simulink model "kurtosis_central_moment_calc"  (R2012b)
settings: Solver=ode45  StartTime=0.0  StopTime=199  RelTol=1e-3
libraries: xbsIndex_r4 x93, simulink_xsg_bridge x1
settings Model: Creator=sgowda  LastModifiedBy=sgowda

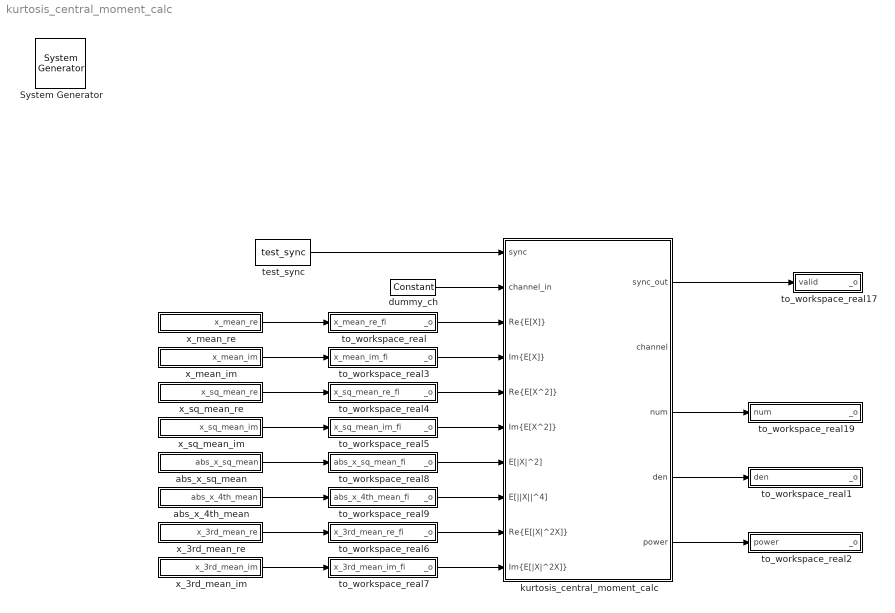
== system kurtosis_central_moment_calc ==
  " System Generator" : xbsIndex_r4/ System Generator  Tag=genX  xilinxfamily=Kintex7  part=xc7k325t  speed=-3  package=fbg676  synthesis_tool=XST  clock_wrapper=Clock Enables  directory=./netlist  proj_type=Project Navigator  Synth_file=XST Defaults  Impl_file=ISE Defaults  testbench=off  simulink_period=1  sysclk_period=10  dcm_input_clock_period=10  incr_netlist=off  trim_vbits=Everywhere in SubSystem  dbl_ovrd=According to Block Masks  core_generation=According to Block Masks  run_coregen=off  deprecated_control=off  eval_field=0  block_type=sysgen
  abs_x_4th_mean : Subsystem  mask{var_name=abs_x_4th_mean, n_bits=88, bin_pt=82, quantization=Round  (unbiased: +/- Inf), overflow=Saturate, arith_type=Signed  (2's comp)}
      mask prompts: var_name "Workspace variable name"; n_bits "# of bits"; bin_pt "Binary Point"; arith_type "Arithmetic type"
      mask init:
      | config.source = str2func('mat_input_data_init_xblock');
      | config.toplevel = gcb();
      | xBlock(config, {config.toplevel, 'var_name', var_name, ...
      |     'n_bits', n_bits, 'bin_pt', bin_pt, 'quantization', quantization, ...
      |     'overflow', overflow, 'arith_type', arith_type});
      mask TypeOptions quantization: Truncate | Round  (unbiased: +/- Inf) | Round  (unbiased: Even Values)
      mask TypeOptions overflow: Wrap | Saturate | Flag as error
      mask TypeOptions arith_type: Signed  (2's comp) | Boolean | Unsigned
  abs_x_sq_mean : Subsystem  mask{var_name=abs_x_sq_mean, n_bits=51, bin_pt=48, quantization=Round  (unbiased: +/- Inf), overflow=Saturate, arith_type=Signed  (2's comp)}
      mask prompts: var_name "Workspace variable name"; n_bits "# of bits"; bin_pt "Binary Point"; arith_type "Arithmetic type"
      mask init: same as kurtosis_central_moment_calc/abs_x_4th_mean
      mask TypeOptions quantization: Truncate | Round  (unbiased: +/- Inf) | Round  (unbiased: Even Values)
      mask TypeOptions overflow: Wrap | Saturate | Flag as error
      mask TypeOptions arith_type: Signed  (2's comp) | Boolean | Unsigned
  dummy_ch : xbsIndex_r4/Constant  const=1  gui_display_data_type=Fixed-point  arith_type=Signed (2's comp)  n_bits=16  bin_pt=14  preci_type=Single  exp_width=8  frac_width=24  explicit_period=on  period=1  equ=P=C  opselect=C  inp2=PCIN>>17  opr=+  inp1=P  carry=CIN  dbl_ovrd=off  block_type=constant
  kurtosis_central_moment_calc : Subsystem
  test_sync : simulink_xsg_bridge/test_sync
  to_workspace_real : Subsystem  mask{var_name=x_mean_re_fi}
      mask prompts: var_name "Workspace variable name"
      mask init:
      | config.source = str2func('mat_output_data_init_xblock');
      | config.toplevel = gcb();
      | xBlock(config, {config.toplevel, 'var_name', var_name});
  to_workspace_real1 : Subsystem  mask{var_name=den}
      mask prompts: var_name "Workspace variable name"
      mask init:
      | config.source = str2func('mat_output_data_init_xblock');
      | config.toplevel = gcb();
      | xBlock(config, {config.toplevel, 'var_name', var_name});
  to_workspace_real17 : Subsystem  mask{var_name=valid}
      mask prompts: var_name "Workspace variable name"
      mask init:
      | config.source = str2func('mat_output_data_init_xblock');
      | config.toplevel = gcb();
      | xBlock(config, {config.toplevel, 'var_name', var_name});
  to_workspace_real19 : Subsystem  mask{var_name=num}
      mask prompts: var_name "Workspace variable name"
      mask init:
      | config.source = str2func('mat_output_data_init_xblock');
      | config.toplevel = gcb();
      | xBlock(config, {config.toplevel, 'var_name', var_name});
  to_workspace_real2 : Subsystem  mask{var_name=power}
      mask prompts: var_name "Workspace variable name"
      mask init:
      | config.source = str2func('mat_output_data_init_xblock');
      | config.toplevel = gcb();
      | xBlock(config, {config.toplevel, 'var_name', var_name});
  to_workspace_real3 : Subsystem  mask{var_name=x_mean_im_fi}
      mask prompts: var_name "Workspace variable name"
      mask init:
      | config.source = str2func('mat_output_data_init_xblock');
      | config.toplevel = gcb();
      | xBlock(config, {config.toplevel, 'var_name', var_name});
  to_workspace_real4 : Subsystem  mask{var_name=x_sq_mean_re_fi}
      mask prompts: var_name "Workspace variable name"
      mask init:
      | config.source = str2func('mat_output_data_init_xblock');
      | config.toplevel = gcb();
      | xBlock(config, {config.toplevel, 'var_name', var_name});
  to_workspace_real5 : Subsystem  mask{var_name=x_sq_mean_im_fi}
      mask prompts: var_name "Workspace variable name"
      mask init:
      | config.source = str2func('mat_output_data_init_xblock');
      | config.toplevel = gcb();
      | xBlock(config, {config.toplevel, 'var_name', var_name});
  to_workspace_real6 : Subsystem  mask{var_name=x_3rd_mean_re_fi}
      mask prompts: var_name "Workspace variable name"
      mask init:
      | config.source = str2func('mat_output_data_init_xblock');
      | config.toplevel = gcb();
      | xBlock(config, {config.toplevel, 'var_name', var_name});
  to_workspace_real7 : Subsystem  mask{var_name=x_3rd_mean_im_fi}
      mask prompts: var_name "Workspace variable name"
      mask init:
      | config.source = str2func('mat_output_data_init_xblock');
      | config.toplevel = gcb();
      | xBlock(config, {config.toplevel, 'var_name', var_name});
  to_workspace_real8 : Subsystem  mask{var_name=abs_x_sq_mean_fi}
      mask prompts: var_name "Workspace variable name"
      mask init:
      | config.source = str2func('mat_output_data_init_xblock');
      | config.toplevel = gcb();
      | xBlock(config, {config.toplevel, 'var_name', var_name});
  to_workspace_real9 : Subsystem  mask{var_name=abs_x_4th_mean_fi}
      mask prompts: var_name "Workspace variable name"
      mask init:
      | config.source = str2func('mat_output_data_init_xblock');
      | config.toplevel = gcb();
      | xBlock(config, {config.toplevel, 'var_name', var_name});
  x_3rd_mean_im : Subsystem  mask{var_name=x_3rd_mean_im, n_bits=69, bin_pt=65, quantization=Round  (unbiased: +/- Inf), overflow=Saturate, arith_type=Signed  (2's comp)}
      mask prompts: var_name "Workspace variable name"; n_bits "# of bits"; bin_pt "Binary Point"; arith_type "Arithmetic type"
      mask init: same as kurtosis_central_moment_calc/abs_x_4th_mean
      mask TypeOptions quantization: Truncate | Round  (unbiased: +/- Inf) | Round  (unbiased: Even Values)
      mask TypeOptions overflow: Wrap | Saturate | Flag as error
      mask TypeOptions arith_type: Signed  (2's comp) | Boolean | Unsigned
  x_3rd_mean_re : Subsystem  mask{var_name=x_3rd_mean_re, n_bits=69, bin_pt=65, quantization=Round  (unbiased: +/- Inf), overflow=Saturate, arith_type=Signed  (2's comp)}
      mask prompts: var_name "Workspace variable name"; n_bits "# of bits"; bin_pt "Binary Point"; arith_type "Arithmetic type"
      mask init: same as kurtosis_central_moment_calc/abs_x_4th_mean
      mask TypeOptions quantization: Truncate | Round  (unbiased: +/- Inf) | Round  (unbiased: Even Values)
      mask TypeOptions overflow: Wrap | Saturate | Flag as error
      mask TypeOptions arith_type: Signed  (2's comp) | Boolean | Unsigned
  x_mean_im : Subsystem  mask{var_name=x_mean_im, n_bits=32, bin_pt=31, quantization=Round  (unbiased: +/- Inf), overflow=Saturate, arith_type=Signed  (2's comp)}
      mask prompts: var_name "Workspace variable name"; n_bits "# of bits"; bin_pt "Binary Point"; arith_type "Arithmetic type"
      mask init: same as kurtosis_central_moment_calc/abs_x_4th_mean
      mask TypeOptions quantization: Truncate | Round  (unbiased: +/- Inf) | Round  (unbiased: Even Values)
      mask TypeOptions overflow: Wrap | Saturate | Flag as error
      mask TypeOptions arith_type: Signed  (2's comp) | Boolean | Unsigned
  x_mean_re : Subsystem  mask{var_name=x_mean_re, n_bits=32, bin_pt=31, quantization=Round  (unbiased: +/- Inf), overflow=Saturate, arith_type=Signed  (2's comp)}
      mask prompts: var_name "Workspace variable name"; n_bits "# of bits"; bin_pt "Binary Point"; arith_type "Arithmetic type"
      mask init: same as kurtosis_central_moment_calc/abs_x_4th_mean
      mask TypeOptions quantization: Truncate | Round  (unbiased: +/- Inf) | Round  (unbiased: Even Values)
      mask TypeOptions overflow: Wrap | Saturate | Flag as error
      mask TypeOptions arith_type: Signed  (2's comp) | Boolean | Unsigned
  x_sq_mean_im : Subsystem  mask{var_name=x_sq_mean_im, n_bits=51, bin_pt=48, quantization=Round  (unbiased: +/- Inf), overflow=Saturate, arith_type=Signed  (2's comp)}
      mask prompts: var_name "Workspace variable name"; n_bits "# of bits"; bin_pt "Binary Point"; arith_type "Arithmetic type"
      mask init: same as kurtosis_central_moment_calc/abs_x_4th_mean
      mask TypeOptions quantization: Truncate | Round  (unbiased: +/- Inf) | Round  (unbiased: Even Values)
      mask TypeOptions overflow: Wrap | Saturate | Flag as error
      mask TypeOptions arith_type: Signed  (2's comp) | Boolean | Unsigned
  x_sq_mean_re : Subsystem  mask{var_name=x_sq_mean_re, n_bits=51, bin_pt=48, quantization=Round  (unbiased: +/- Inf), overflow=Saturate, arith_type=Signed  (2's comp)}
      mask prompts: var_name "Workspace variable name"; n_bits "# of bits"; bin_pt "Binary Point"; arith_type "Arithmetic type"
      mask init: same as kurtosis_central_moment_calc/abs_x_4th_mean
      mask TypeOptions quantization: Truncate | Round  (unbiased: +/- Inf) | Round  (unbiased: Even Values)
      mask TypeOptions overflow: Wrap | Saturate | Flag as error
      mask TypeOptions arith_type: Signed  (2's comp) | Boolean | Unsigned
  wires:
  test_sync/1 -> kurtosis_central_moment_calc/1(sync)
  kurtosis_central_moment_calc/1(sync_out) -> to_workspace_real17/1(valid)
  abs_x_sq_mean/1(abs_x_sq_mean) -> to_workspace_real8/1(abs_x_sq_mean_fi)
  x_mean_im/1(x_mean_im) -> to_workspace_real3/1(x_mean_im_fi)
  x_sq_mean_re/1(x_sq_mean_re) -> to_workspace_real4/1(x_sq_mean_re_fi)
  x_sq_mean_im/1(x_sq_mean_im) -> to_workspace_real5/1(x_sq_mean_im_fi)
  abs_x_4th_mean/1(abs_x_4th_mean) -> to_workspace_real9/1(abs_x_4th_mean_fi)
  x_3rd_mean_re/1(x_3rd_mean_re) -> to_workspace_real6/1(x_3rd_mean_re_fi)
  x_3rd_mean_im/1(x_3rd_mean_im) -> to_workspace_real7/1(x_3rd_mean_im_fi)
  kurtosis_central_moment_calc/3(num) -> to_workspace_real19/1(num)
  kurtosis_central_moment_calc/4(den) -> to_workspace_real1/1(den)
  kurtosis_central_moment_calc/5(power) -> to_workspace_real2/1(power)
  dummy_ch/1 -> kurtosis_central_moment_calc/2(channel_in)
  x_mean_re/1(x_mean_re) -> to_workspace_real/1(x_mean_re_fi)
  to_workspace_real/1(_o) -> kurtosis_central_moment_calc/3("Re{E[X]}")
  to_workspace_real3/1(_o) -> kurtosis_central_moment_calc/4("Im{E[X]}")
  to_workspace_real4/1(_o) -> kurtosis_central_moment_calc/5("Re{E[X^2]}")
  to_workspace_real5/1(_o) -> kurtosis_central_moment_calc/6("Im{E[X^2]}")
  to_workspace_real6/1(_o) -> kurtosis_central_moment_calc/9("Re{E[|X|^2X]}")
  to_workspace_real7/1(_o) -> kurtosis_central_moment_calc/10("Im{E[|X|^2X]}")
  to_workspace_real8/1(_o) -> kurtosis_central_moment_calc/7(E[|X|^2])
  to_workspace_real9/1(_o) -> kurtosis_central_moment_calc/8(E[||X||^4])

== system kurtosis_central_moment_calc/abs_x_4th_mean ==
  gateway : xbsIndex_r4/Gateway In  gui_display_data_type=Fixed-point  arith_type="Signed  (2's comp)"  n_bits=88  bin_pt=82  preci_type=Single  exp_width=8  frac_width=24  quantization="Round  (unbiased: +/- Inf)"  overflow=Saturate  period=1  dbl_ovrd=off  timing_constraint=None  locs_specified=off  LOCs={}  UseAsADC=off  ADCChannel='1'  inherit_from_input=off  hdl_port=on  block_type=gatewayin
  workspace_var : FromWorkspace  VariableName=abs_x_4th_mean  SampleTime=0
  abs_x_4th_mean : Outport
  wires:
  gateway/1 -> abs_x_4th_mean/1
  workspace_var/1 -> gateway/1

== system kurtosis_central_moment_calc/abs_x_sq_mean ==
  gateway : xbsIndex_r4/Gateway In  gui_display_data_type=Fixed-point  arith_type="Signed  (2's comp)"  n_bits=51  bin_pt=48  preci_type=Single  exp_width=8  frac_width=24  quantization="Round  (unbiased: +/- Inf)"  overflow=Saturate  period=1  dbl_ovrd=off  timing_constraint=None  locs_specified=off  LOCs={}  UseAsADC=off  ADCChannel='1'  inherit_from_input=off  hdl_port=on  block_type=gatewayin
  workspace_var : FromWorkspace  VariableName=abs_x_sq_mean  SampleTime=0
  abs_x_sq_mean : Outport
  wires:
  gateway/1 -> abs_x_sq_mean/1
  workspace_var/1 -> gateway/1

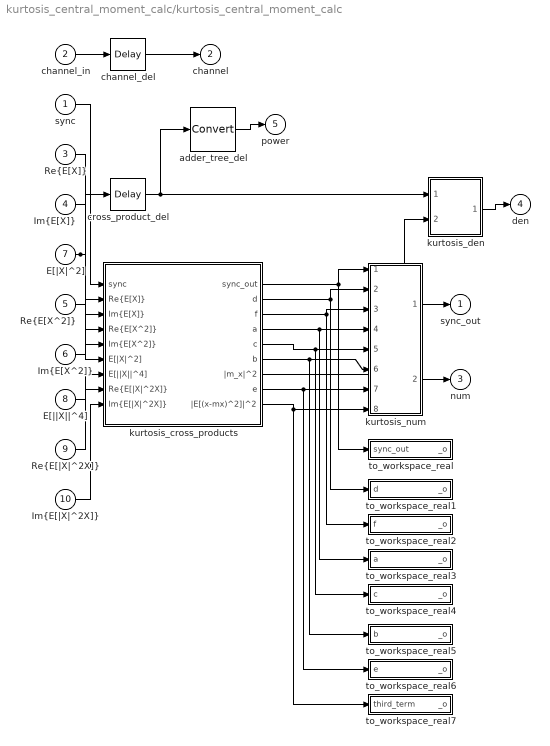
== system kurtosis_central_moment_calc/kurtosis_central_moment_calc ==
  sync : Inport
  channel_in : Inport  Port=2
  "Re{E[X]}" : Inport  Port=3
  "Im{E[X]}" : Inport  Port=4
  "Re{E[X^2]}" : Inport  Port=5
  "Im{E[X^2]}" : Inport  Port=6
  E[|X|^2] : Inport  Port=7
  E[||X||^4] : Inport  Port=8
  "Re{E[|X|^2X]}" : Inport  Port=9
  "Im{E[|X|^2X]}" : Inport  Port=10
  adder_tree_del : xbsIndex_r4/Convert  gui_display_data_type=Fixed-point  arith_type="Signed  (2's comp)"  n_bits=32  bin_pt=29  float_type=Single  exp_bits=8  fraction_bits=24  quantization="Round  (unbiased: +/- Inf)"  overflow=Saturate  en=off  latency=13  dbl_ovrd=off  pipeline=off  block_type=convert
  channel_del : xbsIndex_r4/Delay  rst=off  infoeditControl=Selection of Reset will increase slice count due to use of real FFs and instead of SRLs  en=off  latency=38  dbl_ovrd=off  reg_retiming=off  block_type=delay
  cross_product_del : xbsIndex_r4/Delay  rst=off  infoeditControl=Selection of Reset will increase slice count due to use of real FFs and instead of SRLs  en=off  latency=25  dbl_ovrd=off  reg_retiming=off  block_type=delay
  kurtosis_cross_products : Subsystem
  kurtosis_den : Subsystem
  kurtosis_num : Subsystem
  to_workspace_real : Subsystem  mask{var_name=sync_out}
      mask prompts: var_name "Workspace variable name"
      mask init:
      | config.source = str2func('mat_output_data_init_xblock');
      | config.toplevel = gcb();
      | xBlock(config, {config.toplevel, 'var_name', var_name});
  to_workspace_real1 : Subsystem  mask{var_name=d}
      mask prompts: var_name "Workspace variable name"
      mask init:
      | config.source = str2func('mat_output_data_init_xblock');
      | config.toplevel = gcb();
      | xBlock(config, {config.toplevel, 'var_name', var_name});
  to_workspace_real2 : Subsystem  mask{var_name=f}
      mask prompts: var_name "Workspace variable name"
      mask init:
      | config.source = str2func('mat_output_data_init_xblock');
      | config.toplevel = gcb();
      | xBlock(config, {config.toplevel, 'var_name', var_name});
  to_workspace_real3 : Subsystem  mask{var_name=a}
      mask prompts: var_name "Workspace variable name"
      mask init:
      | config.source = str2func('mat_output_data_init_xblock');
      | config.toplevel = gcb();
      | xBlock(config, {config.toplevel, 'var_name', var_name});
  to_workspace_real4 : Subsystem  mask{var_name=c}
      mask prompts: var_name "Workspace variable name"
      mask init:
      | config.source = str2func('mat_output_data_init_xblock');
      | config.toplevel = gcb();
      | xBlock(config, {config.toplevel, 'var_name', var_name});
  to_workspace_real5 : Subsystem  mask{var_name=b}
      mask prompts: var_name "Workspace variable name"
      mask init:
      | config.source = str2func('mat_output_data_init_xblock');
      | config.toplevel = gcb();
      | xBlock(config, {config.toplevel, 'var_name', var_name});
  to_workspace_real6 : Subsystem  mask{var_name=e}
      mask prompts: var_name "Workspace variable name"
      mask init:
      | config.source = str2func('mat_output_data_init_xblock');
      | config.toplevel = gcb();
      | xBlock(config, {config.toplevel, 'var_name', var_name});
  to_workspace_real7 : Subsystem  mask{var_name=third_term}
      mask prompts: var_name "Workspace variable name"
      mask init:
      | config.source = str2func('mat_output_data_init_xblock');
      | config.toplevel = gcb();
      | xBlock(config, {config.toplevel, 'var_name', var_name});
  sync_out : Outport
  channel : Outport  Port=2
  num : Outport  Port=3
  den : Outport  Port=4
  power : Outport  Port=5
  wires:
  E[|X|^2]/1 -> kurtosis_cross_products/6(E[|X|^2]), cross_product_del/1
  cross_product_del/1 -> kurtosis_den/1(E[|X|^2]), adder_tree_del/1
  channel_del/1 -> channel/1
  channel_in/1 -> channel_del/1
  kurtosis_num/2(E[|X-m_x|^4]) -> num/1
  kurtosis_num/1(sync_out) -> sync_out/1
  kurtosis_cross_products/9(|E[(x-mx)^2]|^2) -> to_workspace_real7/1(third_term), kurtosis_num/8(|E[(x-mx)^2]|^2)
  kurtosis_cross_products/8(e) -> to_workspace_real6/1(e), kurtosis_num/7(|m_x|^4)
  kurtosis_cross_products/6(b) -> to_workspace_real5/1(b), kurtosis_num/6("Re{4E[X|X|^2*m_x]}")
  kurtosis_cross_products/5(c) -> to_workspace_real4/1(c), kurtosis_num/5("Re{2E[X^2*conj(m_x^2)]}")
  kurtosis_cross_products/4(a) -> to_workspace_real3/1(a), kurtosis_num/4(E[|X|^4])
  kurtosis_cross_products/3(f) -> kurtosis_num/3(4|m_x|^4), to_workspace_real2/1(f)
  kurtosis_cross_products/2(d) -> kurtosis_num/2(4E[|X|^2]|m_x|^2), to_workspace_real1/1(d)
  kurtosis_cross_products/1(sync_out) -> kurtosis_num/1(sync), to_workspace_real/1(sync_out)
  kurtosis_den/1(E[|X-m_x|^2]^2) -> den/1
  kurtosis_cross_products/7(|m_x|^2) -> kurtosis_den/2(|m_x|^2)
  "Im{E[|X|^2X]}"/1 -> kurtosis_cross_products/9("Im{E[|X|^2X]}")
  "Re{E[|X|^2X]}"/1 -> kurtosis_cross_products/8("Re{E[|X|^2X]}")
  E[||X||^4]/1 -> kurtosis_cross_products/7(E[||X||^4])
  "Im{E[X^2]}"/1 -> kurtosis_cross_products/5("Im{E[X^2]}")
  "Re{E[X^2]}"/1 -> kurtosis_cross_products/4("Re{E[X^2]}")
  "Im{E[X]}"/1 -> kurtosis_cross_products/3("Im{E[X]}")
  "Re{E[X]}"/1 -> kurtosis_cross_products/2("Re{E[X]}")
  sync/1 -> kurtosis_cross_products/1(sync)
  adder_tree_del/1 -> power/1

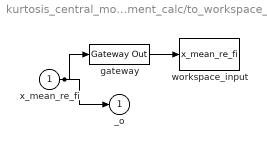
== system kurtosis_central_moment_calc/to_workspace_real ==
  x_mean_re_fi : Inport
  gateway : xbsIndex_r4/Gateway Out  inherit_from_input=on  hdl_port=off  timing_constraint=None  locs_specified=off  LOCs={}  UseAsDAC=off  DACChannel='1'  block_type=gatewayout
  workspace_input : ToWorkspace  VariableName=x_mean_re_fi  SampleTime=-1
  _o : Outport
  wires:
  x_mean_re_fi/1 -> gateway/1, _o/1
  gateway/1 -> workspace_input/1

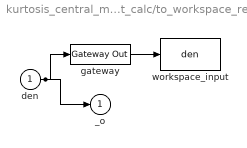
== system kurtosis_central_moment_calc/to_workspace_real1 ==
  den : Inport
  gateway : xbsIndex_r4/Gateway Out  inherit_from_input=on  hdl_port=off  timing_constraint=None  locs_specified=off  LOCs={}  UseAsDAC=off  DACChannel='1'  block_type=gatewayout
  workspace_input : ToWorkspace  VariableName=den  SampleTime=-1
  _o : Outport
  wires:
  den/1 -> gateway/1, _o/1
  gateway/1 -> workspace_input/1

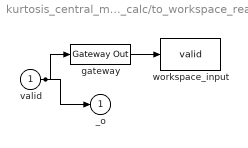
== system kurtosis_central_moment_calc/to_workspace_real17 ==
  valid : Inport
  gateway : xbsIndex_r4/Gateway Out  inherit_from_input=on  hdl_port=off  timing_constraint=None  locs_specified=off  LOCs={}  UseAsDAC=off  DACChannel='1'  block_type=gatewayout
  workspace_input : ToWorkspace  VariableName=valid  SampleTime=-1
  _o : Outport
  wires:
  valid/1 -> gateway/1, _o/1
  gateway/1 -> workspace_input/1

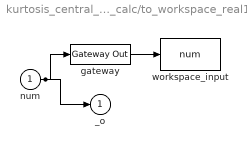
== system kurtosis_central_moment_calc/to_workspace_real19 ==
  num : Inport
  gateway : xbsIndex_r4/Gateway Out  inherit_from_input=on  hdl_port=off  timing_constraint=None  locs_specified=off  LOCs={}  UseAsDAC=off  DACChannel='1'  block_type=gatewayout
  workspace_input : ToWorkspace  VariableName=num  SampleTime=-1
  _o : Outport
  wires:
  num/1 -> gateway/1, _o/1
  gateway/1 -> workspace_input/1

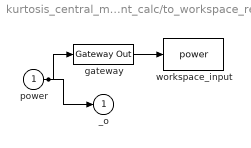
== system kurtosis_central_moment_calc/to_workspace_real2 ==
  power : Inport
  gateway : xbsIndex_r4/Gateway Out  inherit_from_input=on  hdl_port=off  timing_constraint=None  locs_specified=off  LOCs={}  UseAsDAC=off  DACChannel='1'  block_type=gatewayout
  workspace_input : ToWorkspace  VariableName=power  SampleTime=-1
  _o : Outport
  wires:
  power/1 -> gateway/1, _o/1
  gateway/1 -> workspace_input/1

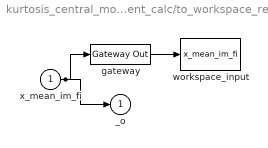
== system kurtosis_central_moment_calc/to_workspace_real3 ==
  x_mean_im_fi : Inport
  gateway : xbsIndex_r4/Gateway Out  inherit_from_input=on  hdl_port=off  timing_constraint=None  locs_specified=off  LOCs={}  UseAsDAC=off  DACChannel='1'  block_type=gatewayout
  workspace_input : ToWorkspace  VariableName=x_mean_im_fi  SampleTime=-1
  _o : Outport
  wires:
  x_mean_im_fi/1 -> gateway/1, _o/1
  gateway/1 -> workspace_input/1

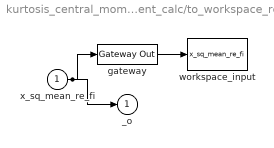
== system kurtosis_central_moment_calc/to_workspace_real4 ==
  x_sq_mean_re_fi : Inport
  gateway : xbsIndex_r4/Gateway Out  inherit_from_input=on  hdl_port=off  timing_constraint=None  locs_specified=off  LOCs={}  UseAsDAC=off  DACChannel='1'  block_type=gatewayout
  workspace_input : ToWorkspace  VariableName=x_sq_mean_re_fi  SampleTime=-1
  _o : Outport
  wires:
  x_sq_mean_re_fi/1 -> gateway/1, _o/1
  gateway/1 -> workspace_input/1

== system kurtosis_central_moment_calc/to_workspace_real5 ==
  x_sq_mean_im_fi : Inport
  gateway : xbsIndex_r4/Gateway Out  inherit_from_input=on  hdl_port=off  timing_constraint=None  locs_specified=off  LOCs={}  UseAsDAC=off  DACChannel='1'  block_type=gatewayout
  workspace_input : ToWorkspace  VariableName=x_sq_mean_im_fi  SampleTime=-1
  _o : Outport
  wires:
  x_sq_mean_im_fi/1 -> gateway/1, _o/1
  gateway/1 -> workspace_input/1

== system kurtosis_central_moment_calc/to_workspace_real6 ==
  x_3rd_mean_re_fi : Inport
  gateway : xbsIndex_r4/Gateway Out  inherit_from_input=on  hdl_port=off  timing_constraint=None  locs_specified=off  LOCs={}  UseAsDAC=off  DACChannel='1'  block_type=gatewayout
  workspace_input : ToWorkspace  VariableName=x_3rd_mean_re_fi  SampleTime=-1
  _o : Outport
  wires:
  x_3rd_mean_re_fi/1 -> gateway/1, _o/1
  gateway/1 -> workspace_input/1

== system kurtosis_central_moment_calc/to_workspace_real7 ==
  x_3rd_mean_im_fi : Inport
  gateway : xbsIndex_r4/Gateway Out  inherit_from_input=on  hdl_port=off  timing_constraint=None  locs_specified=off  LOCs={}  UseAsDAC=off  DACChannel='1'  block_type=gatewayout
  workspace_input : ToWorkspace  VariableName=x_3rd_mean_im_fi  SampleTime=-1
  _o : Outport
  wires:
  x_3rd_mean_im_fi/1 -> gateway/1, _o/1
  gateway/1 -> workspace_input/1

== system kurtosis_central_moment_calc/to_workspace_real8 ==
  abs_x_sq_mean_fi : Inport
  gateway : xbsIndex_r4/Gateway Out  inherit_from_input=on  hdl_port=off  timing_constraint=None  locs_specified=off  LOCs={}  UseAsDAC=off  DACChannel='1'  block_type=gatewayout
  workspace_input : ToWorkspace  VariableName=abs_x_sq_mean_fi  SampleTime=-1
  _o : Outport
  wires:
  abs_x_sq_mean_fi/1 -> gateway/1, _o/1
  gateway/1 -> workspace_input/1

== system kurtosis_central_moment_calc/to_workspace_real9 ==
  abs_x_4th_mean_fi : Inport
  gateway : xbsIndex_r4/Gateway Out  inherit_from_input=on  hdl_port=off  timing_constraint=None  locs_specified=off  LOCs={}  UseAsDAC=off  DACChannel='1'  block_type=gatewayout
  workspace_input : ToWorkspace  VariableName=abs_x_4th_mean_fi  SampleTime=-1
  _o : Outport
  wires:
  abs_x_4th_mean_fi/1 -> gateway/1, _o/1
  gateway/1 -> workspace_input/1

== system kurtosis_central_moment_calc/x_3rd_mean_im ==
  gateway : xbsIndex_r4/Gateway In  gui_display_data_type=Fixed-point  arith_type="Signed  (2's comp)"  n_bits=69  bin_pt=65  preci_type=Single  exp_width=8  frac_width=24  quantization="Round  (unbiased: +/- Inf)"  overflow=Saturate  period=1  dbl_ovrd=off  timing_constraint=None  locs_specified=off  LOCs={}  UseAsADC=off  ADCChannel='1'  inherit_from_input=off  hdl_port=on  block_type=gatewayin
  workspace_var : FromWorkspace  VariableName=x_3rd_mean_im  SampleTime=0
  x_3rd_mean_im : Outport
  wires:
  gateway/1 -> x_3rd_mean_im/1
  workspace_var/1 -> gateway/1

== system kurtosis_central_moment_calc/x_3rd_mean_re ==
  gateway : xbsIndex_r4/Gateway In  gui_display_data_type=Fixed-point  arith_type="Signed  (2's comp)"  n_bits=69  bin_pt=65  preci_type=Single  exp_width=8  frac_width=24  quantization="Round  (unbiased: +/- Inf)"  overflow=Saturate  period=1  dbl_ovrd=off  timing_constraint=None  locs_specified=off  LOCs={}  UseAsADC=off  ADCChannel='1'  inherit_from_input=off  hdl_port=on  block_type=gatewayin
  workspace_var : FromWorkspace  VariableName=x_3rd_mean_re  SampleTime=0
  x_3rd_mean_re : Outport
  wires:
  gateway/1 -> x_3rd_mean_re/1
  workspace_var/1 -> gateway/1

== system kurtosis_central_moment_calc/x_mean_im ==
  gateway : xbsIndex_r4/Gateway In  gui_display_data_type=Fixed-point  arith_type="Signed  (2's comp)"  n_bits=32  bin_pt=31  preci_type=Single  exp_width=8  frac_width=24  quantization="Round  (unbiased: +/- Inf)"  overflow=Saturate  period=1  dbl_ovrd=off  timing_constraint=None  locs_specified=off  LOCs={}  UseAsADC=off  ADCChannel='1'  inherit_from_input=off  hdl_port=on  block_type=gatewayin
  workspace_var : FromWorkspace  VariableName=x_mean_im  SampleTime=0
  x_mean_im : Outport
  wires:
  gateway/1 -> x_mean_im/1
  workspace_var/1 -> gateway/1

== system kurtosis_central_moment_calc/x_mean_re ==
  gateway : xbsIndex_r4/Gateway In  gui_display_data_type=Fixed-point  arith_type="Signed  (2's comp)"  n_bits=32  bin_pt=31  preci_type=Single  exp_width=8  frac_width=24  quantization="Round  (unbiased: +/- Inf)"  overflow=Saturate  period=1  dbl_ovrd=off  timing_constraint=None  locs_specified=off  LOCs={}  UseAsADC=off  ADCChannel='1'  inherit_from_input=off  hdl_port=on  block_type=gatewayin
  workspace_var : FromWorkspace  VariableName=x_mean_re  SampleTime=0
  x_mean_re : Outport
  wires:
  gateway/1 -> x_mean_re/1
  workspace_var/1 -> gateway/1

== system kurtosis_central_moment_calc/x_sq_mean_im ==
  gateway : xbsIndex_r4/Gateway In  gui_display_data_type=Fixed-point  arith_type="Signed  (2's comp)"  n_bits=51  bin_pt=48  preci_type=Single  exp_width=8  frac_width=24  quantization="Round  (unbiased: +/- Inf)"  overflow=Saturate  period=1  dbl_ovrd=off  timing_constraint=None  locs_specified=off  LOCs={}  UseAsADC=off  ADCChannel='1'  inherit_from_input=off  hdl_port=on  block_type=gatewayin
  workspace_var : FromWorkspace  VariableName=x_sq_mean_im  SampleTime=0
  x_sq_mean_im : Outport
  wires:
  gateway/1 -> x_sq_mean_im/1
  workspace_var/1 -> gateway/1

== system kurtosis_central_moment_calc/x_sq_mean_re ==
  gateway : xbsIndex_r4/Gateway In  gui_display_data_type=Fixed-point  arith_type="Signed  (2's comp)"  n_bits=51  bin_pt=48  preci_type=Single  exp_width=8  frac_width=24  quantization="Round  (unbiased: +/- Inf)"  overflow=Saturate  period=1  dbl_ovrd=off  timing_constraint=None  locs_specified=off  LOCs={}  UseAsADC=off  ADCChannel='1'  inherit_from_input=off  hdl_port=on  block_type=gatewayin
  workspace_var : FromWorkspace  VariableName=x_sq_mean_re  SampleTime=0
  x_sq_mean_re : Outport
  wires:
  gateway/1 -> x_sq_mean_re/1
  workspace_var/1 -> gateway/1

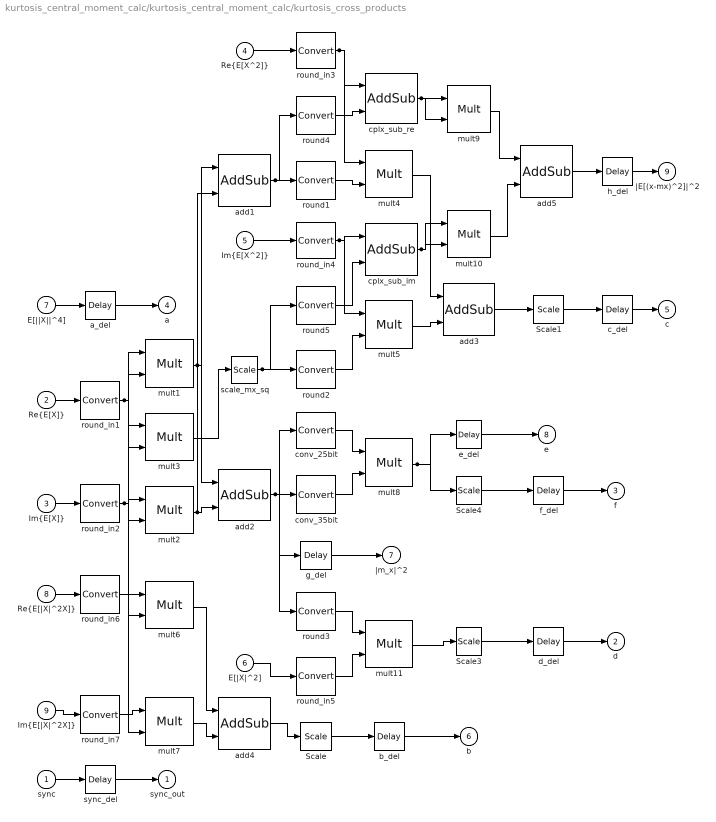
== system kurtosis_central_moment_calc/kurtosis_central_moment_calc/kurtosis_cross_products ==
  sync : Inport
  "Re{E[X]}" : Inport  Port=2
  "Im{E[X]}" : Inport  Port=3
  "Re{E[X^2]}" : Inport  Port=4
  "Im{E[X^2]}" : Inport  Port=5
  E[|X|^2] : Inport  Port=6
  E[||X||^4] : Inport  Port=7
  "Re{E[|X|^2X]}" : Inport  Port=8
  "Im{E[|X|^2X]}" : Inport  Port=9
  Scale : xbsIndex_r4/Scale  scale_factor=2  dbl_ovrd=off  block_type=scale
  Scale1 : xbsIndex_r4/Scale  scale_factor=1  dbl_ovrd=off  block_type=scale
  Scale3 : xbsIndex_r4/Scale  scale_factor=2  dbl_ovrd=off  block_type=scale
  Scale4 : xbsIndex_r4/Scale  scale_factor=2  dbl_ovrd=off  block_type=scale
  a_del : xbsIndex_r4/Delay  rst=off  infoeditControl=Selection of Reset will increase slice count due to use of real FFs and instead of SRLs  en=off  latency=25  dbl_ovrd=off  reg_retiming=off  block_type=delay
  add1 : xbsIndex_r4/AddSub  mode=Subtraction  use_carryin=off  use_carryout=off  en=off  latency=2  precision=Full  arith_type="Signed  (2's comp)"  n_bits=36  bin_pt=34  quantization=Truncate  overflow=Wrap  dbl_ovrd=off  use_behavioral_HDL=off  hw_selection=Fabric  pipelined=off  block_type=addsub
  add2 : xbsIndex_r4/AddSub  mode=Addition  use_carryin=off  use_carryout=off  en=off  latency=2  precision=Full  arith_type="Signed  (2's comp)"  n_bits=36  bin_pt=34  quantization=Truncate  overflow=Wrap  dbl_ovrd=off  use_behavioral_HDL=off  hw_selection=Fabric  pipelined=off  block_type=addsub
  add3 : xbsIndex_r4/AddSub  mode=Addition  use_carryin=off  use_carryout=off  en=off  latency=3  precision=Full  arith_type="Signed  (2's comp)"  n_bits=36  bin_pt=34  quantization=Truncate  overflow=Wrap  dbl_ovrd=off  use_behavioral_HDL=off  hw_selection=Fabric  pipelined=off  block_type=addsub
  add4 : xbsIndex_r4/AddSub  mode=Addition  use_carryin=off  use_carryout=off  en=off  latency=3  precision=Full  arith_type="Signed  (2's comp)"  n_bits=36  bin_pt=34  quantization=Truncate  overflow=Wrap  dbl_ovrd=off  use_behavioral_HDL=off  hw_selection=Fabric  pipelined=off  block_type=addsub
  add5 : xbsIndex_r4/AddSub  mode=Addition  use_carryin=off  use_carryout=off  en=off  latency=3  precision=Full  arith_type="Signed  (2's comp)"  n_bits=36  bin_pt=34  quantization=Truncate  overflow=Wrap  dbl_ovrd=off  use_behavioral_HDL=off  hw_selection=Fabric  pipelined=off  block_type=addsub
  b_del : xbsIndex_r4/Delay  rst=off  infoeditControl=Selection of Reset will increase slice count due to use of real FFs and instead of SRLs  en=off  latency=15  dbl_ovrd=off  reg_retiming=off  block_type=delay
  c_del : xbsIndex_r4/Delay  rst=off  infoeditControl=Selection of Reset will increase slice count due to use of real FFs and instead of SRLs  en=off  latency=6  dbl_ovrd=off  reg_retiming=off  block_type=delay
  conv_25bit : xbsIndex_r4/Convert  gui_display_data_type=Fixed-point  arith_type="Signed  (2's comp)"  n_bits=25  bin_pt=22  float_type=Single  exp_bits=8  fraction_bits=24  quantization="Round  (unbiased: +/- Inf)"  overflow=Saturate  en=off  latency=3  dbl_ovrd=off  pipeline=off  block_type=convert
  conv_35bit : xbsIndex_r4/Convert  gui_display_data_type=Fixed-point  arith_type="Signed  (2's comp)"  n_bits=35  bin_pt=32  float_type=Single  exp_bits=8  fraction_bits=24  quantization="Round  (unbiased: +/- Inf)"  overflow=Saturate  en=off  latency=3  dbl_ovrd=off  pipeline=off  block_type=convert
  cplx_sub_im : xbsIndex_r4/AddSub  mode=Subtraction  use_carryin=off  use_carryout=off  en=off  latency=2  precision=Full  arith_type="Signed  (2's comp)"  n_bits=36  bin_pt=34  quantization=Truncate  overflow=Wrap  dbl_ovrd=off  use_behavioral_HDL=off  hw_selection=Fabric  pipelined=off  block_type=addsub
  cplx_sub_re : xbsIndex_r4/AddSub  mode=Subtraction  use_carryin=off  use_carryout=off  en=off  latency=2  precision=Full  arith_type="Signed  (2's comp)"  n_bits=36  bin_pt=34  quantization=Truncate  overflow=Wrap  dbl_ovrd=off  use_behavioral_HDL=off  hw_selection=Fabric  pipelined=off  block_type=addsub
  d_del : xbsIndex_r4/Delay  rst=off  infoeditControl=Selection of Reset will increase slice count due to use of real FFs and instead of SRLs  en=off  latency=9  dbl_ovrd=off  reg_retiming=off  block_type=delay
  e_del : xbsIndex_r4/Delay  rst=off  infoeditControl=Selection of Reset will increase slice count due to use of real FFs and instead of SRLs  en=off  latency=9  dbl_ovrd=off  reg_retiming=off  block_type=delay
  f_del : xbsIndex_r4/Delay  rst=off  infoeditControl=Selection of Reset will increase slice count due to use of real FFs and instead of SRLs  en=off  latency=9  dbl_ovrd=off  reg_retiming=off  block_type=delay
  g_del : xbsIndex_r4/Delay  rst=off  infoeditControl=Selection of Reset will increase slice count due to use of real FFs and instead of SRLs  en=off  latency=16  dbl_ovrd=off  reg_retiming=off  block_type=delay
  h_del : xbsIndex_r4/Delay  rst=off  infoeditControl=Selection of Reset will increase slice count due to use of real FFs and instead of SRLs  en=off  latency=2  dbl_ovrd=off  reg_retiming=off  block_type=delay
  mult{1..8,11} (9 alike) : xbsIndex_r4/Mult  precision=Full  arith_type="Signed  (2's comp)"  n_bits=36  bin_pt=34  quantization=Truncate  overflow=Wrap  en=off  latency=4  dbl_ovrd=off  use_behavioral_HDL=off  opt=Speed  use_embedded=on  optimum_pipeline=off  pipeline=on  use_rpm=on  placement_style=Triangular  block_type=mult
  mult10 : xbsIndex_r4/Mult  precision=Full  arith_type="Signed  (2's comp)"  n_bits=36  bin_pt=34  quantization=Truncate  overflow=Wrap  en=off  latency=6  dbl_ovrd=off  use_behavioral_HDL=off  opt=Speed  use_embedded=on  optimum_pipeline=off  pipeline=on  use_rpm=on  placement_style=Triangular  block_type=mult
  mult9 : xbsIndex_r4/Mult  precision=Full  arith_type="Signed  (2's comp)"  n_bits=36  bin_pt=34  quantization=Truncate  overflow=Wrap  en=off  latency=6  dbl_ovrd=off  use_behavioral_HDL=off  opt=Speed  use_embedded=on  optimum_pipeline=off  pipeline=on  use_rpm=on  placement_style=Triangular  block_type=mult
  round1 : xbsIndex_r4/Convert  gui_display_data_type=Fixed-point  arith_type="Signed  (2's comp)"  n_bits=25  bin_pt=22  float_type=Single  exp_bits=8  fraction_bits=24  quantization="Round  (unbiased: +/- Inf)"  overflow=Saturate  en=off  latency=3  dbl_ovrd=off  pipeline=off  block_type=convert
  round2 : xbsIndex_r4/Convert  gui_display_data_type=Fixed-point  arith_type="Signed  (2's comp)"  n_bits=25  bin_pt=22  float_type=Single  exp_bits=8  fraction_bits=24  quantization="Round  (unbiased: +/- Inf)"  overflow=Saturate  en=off  latency=5  dbl_ovrd=off  pipeline=off  block_type=convert
  round3 : xbsIndex_r4/Convert  gui_display_data_type=Fixed-point  arith_type="Signed  (2's comp)"  n_bits=25  bin_pt=22  float_type=Single  exp_bits=8  fraction_bits=24  quantization="Round  (unbiased: +/- Inf)"  overflow=Saturate  en=off  latency=3  dbl_ovrd=off  pipeline=off  block_type=convert
  round4 : xbsIndex_r4/Convert  gui_display_data_type=Fixed-point  arith_type="Signed  (2's comp)"  n_bits=35  bin_pt=32  float_type=Single  exp_bits=8  fraction_bits=24  quantization="Round  (unbiased: +/- Inf)"  overflow=Saturate  en=off  latency=3  dbl_ovrd=off  pipeline=off  block_type=convert
  round5 : xbsIndex_r4/Convert  gui_display_data_type=Fixed-point  arith_type="Signed  (2's comp)"  n_bits=35  bin_pt=32  float_type=Single  exp_bits=8  fraction_bits=24  quantization="Round  (unbiased: +/- Inf)"  overflow=Saturate  en=off  latency=3  dbl_ovrd=off  pipeline=off  block_type=convert
  round_in1 : xbsIndex_r4/Convert  gui_display_data_type=Fixed-point  arith_type="Signed  (2's comp)"  n_bits=25  bin_pt=24  float_type=Single  exp_bits=8  fraction_bits=24  quantization="Round  (unbiased: +/- Inf)"  overflow=Saturate  en=off  latency=3  dbl_ovrd=off  pipeline=off  block_type=convert
  round_in2 : xbsIndex_r4/Convert  gui_display_data_type=Fixed-point  arith_type="Signed  (2's comp)"  n_bits=25  bin_pt=24  float_type=Single  exp_bits=8  fraction_bits=24  quantization="Round  (unbiased: +/- Inf)"  overflow=Saturate  en=off  latency=3  dbl_ovrd=off  pipeline=off  block_type=convert
  round_in3 : xbsIndex_r4/Convert  gui_display_data_type=Fixed-point  arith_type="Signed  (2's comp)"  n_bits=35  bin_pt=32  float_type=Single  exp_bits=8  fraction_bits=24  quantization="Round  (unbiased: +/- Inf)"  overflow=Saturate  en=off  latency=12  dbl_ovrd=off  pipeline=off  block_type=convert
  round_in4 : xbsIndex_r4/Convert  gui_display_data_type=Fixed-point  arith_type="Signed  (2's comp)"  n_bits=35  bin_pt=32  float_type=Single  exp_bits=8  fraction_bits=24  quantization="Round  (unbiased: +/- Inf)"  overflow=Saturate  en=off  latency=12  dbl_ovrd=off  pipeline=off  block_type=convert
  round_in5 : xbsIndex_r4/Convert  gui_display_data_type=Fixed-point  arith_type="Signed  (2's comp)"  n_bits=35  bin_pt=32  float_type=Single  exp_bits=8  fraction_bits=24  quantization="Round  (unbiased: +/- Inf)"  overflow=Saturate  en=off  latency=12  dbl_ovrd=off  pipeline=off  block_type=convert
  round_in6 : xbsIndex_r4/Convert  gui_display_data_type=Fixed-point  arith_type="Signed  (2's comp)"  n_bits=35  bin_pt=31  float_type=Single  exp_bits=8  fraction_bits=24  quantization="Round  (unbiased: +/- Inf)"  overflow=Saturate  en=off  latency=3  dbl_ovrd=off  pipeline=off  block_type=convert
  round_in7 : xbsIndex_r4/Convert  gui_display_data_type=Fixed-point  arith_type="Signed  (2's comp)"  n_bits=35  bin_pt=31  float_type=Single  exp_bits=8  fraction_bits=24  quantization="Round  (unbiased: +/- Inf)"  overflow=Saturate  en=off  latency=3  dbl_ovrd=off  pipeline=off  block_type=convert
  scale_mx_sq : xbsIndex_r4/Scale  scale_factor=1  dbl_ovrd=off  block_type=scale
  sync_del : xbsIndex_r4/Delay  rst=off  infoeditControl=Selection of Reset will increase slice count due to use of real FFs and instead of SRLs  en=off  latency=25  dbl_ovrd=off  reg_retiming=off  block_type=delay
  sync_out : Outport
  d : Outport  Port=2
  f : Outport  Port=3
  a : Outport  Port=4
  c : Outport  Port=5
  b : Outport  Port=6
  |m_x|^2 : Outport  Port=7
  e : Outport  Port=8
  |E[(x-mx)^2]|^2 : Outport  Port=9
  wires:
  round_in1/1 -> mult6/2, mult3/1, mult1/2, mult1/1
  round_in2/1 -> mult7/2, mult3/2, mult2/2, mult2/1
  mult1/1 -> add2/1, add1/1
  mult2/1 -> add2/2, add1/2
  add1/1 -> round4/1, round1/1
  scale_mx_sq/1 -> round5/1, round2/1
  round_in3/1 -> cplx_sub_re/1, mult4/1
  round_in4/1 -> cplx_sub_im/1, mult5/1
  add2/1 -> g_del/1, round3/1, conv_35bit/1, conv_25bit/1
  mult8/1 -> e_del/1, Scale4/1
  cplx_sub_re/1 -> mult9/2, mult9/1
  cplx_sub_im/1 -> mult10/2, mult10/1
  h_del/1 -> |E[(x-mx)^2]|^2/1
  g_del/1 -> |m_x|^2/1
  f_del/1 -> f/1
  e_del/1 -> e/1
  d_del/1 -> d/1
  c_del/1 -> c/1
  b_del/1 -> b/1
  a_del/1 -> a/1
  sync_del/1 -> sync_out/1
  sync/1 -> sync_del/1
  add5/1 -> h_del/1
  Scale4/1 -> f_del/1
  Scale3/1 -> d_del/1
  Scale1/1 -> c_del/1
  Scale/1 -> b_del/1
  E[||X||^4]/1 -> a_del/1
  mult10/1 -> add5/2
  mult9/1 -> add5/1
  round5/1 -> cplx_sub_im/2
  round4/1 -> cplx_sub_re/2
  mult11/1 -> Scale3/1
  round_in5/1 -> mult11/2
  round3/1 -> mult11/1
  conv_35bit/1 -> mult8/2
  conv_25bit/1 -> mult8/1
  add4/1 -> Scale/1
  mult7/1 -> add4/2
  mult6/1 -> add4/1
  round_in7/1 -> mult7/1
  round_in6/1 -> mult6/1
  add3/1 -> Scale1/1
  mult5/1 -> add3/2
  mult4/1 -> add3/1
  round2/1 -> mult5/2
  round1/1 -> mult4/2
  mult3/1 -> scale_mx_sq/1
  "Im{E[|X|^2X]}"/1 -> round_in7/1
  "Re{E[|X|^2X]}"/1 -> round_in6/1
  E[|X|^2]/1 -> round_in5/1
  "Im{E[X^2]}"/1 -> round_in4/1
  "Re{E[X^2]}"/1 -> round_in3/1
  "Im{E[X]}"/1 -> round_in2/1
  "Re{E[X]}"/1 -> round_in1/1

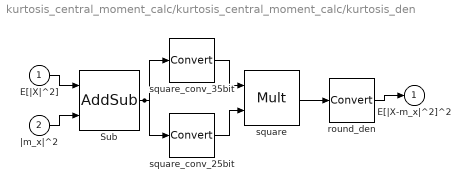
== system kurtosis_central_moment_calc/kurtosis_central_moment_calc/kurtosis_den ==
  E[|X|^2] : Inport
  |m_x|^2 : Inport  Port=2
  Sub : xbsIndex_r4/AddSub  mode=Subtraction  use_carryin=off  use_carryout=off  en=off  latency=4  precision=Full  arith_type="Signed  (2's comp)"  n_bits=36  bin_pt=34  quantization=Truncate  overflow=Wrap  dbl_ovrd=off  use_behavioral_HDL=off  hw_selection=Fabric  pipelined=off  block_type=addsub
  round_den : xbsIndex_r4/Convert  gui_display_data_type=Fixed-point  arith_type="Signed  (2's comp)"  n_bits=64  bin_pt=56  float_type=Single  exp_bits=8  fraction_bits=24  quantization="Round  (unbiased: +/- Inf)"  overflow=Saturate  en=off  latency=1  dbl_ovrd=off  pipeline=off  block_type=convert
  square : xbsIndex_r4/Mult  precision=Full  arith_type="Signed  (2's comp)"  n_bits=36  bin_pt=34  quantization=Truncate  overflow=Wrap  en=off  latency=5  dbl_ovrd=off  use_behavioral_HDL=off  opt=Speed  use_embedded=on  optimum_pipeline=off  pipeline=on  use_rpm=on  placement_style=Triangular  block_type=mult
  square_conv_25bit : xbsIndex_r4/Convert  gui_display_data_type=Fixed-point  arith_type="Signed  (2's comp)"  n_bits=25  bin_pt=21  float_type=Single  exp_bits=8  fraction_bits=24  quantization="Round  (unbiased: +/- Inf)"  overflow=Saturate  en=off  latency=3  dbl_ovrd=off  pipeline=off  block_type=convert
  square_conv_35bit : xbsIndex_r4/Convert  gui_display_data_type=Fixed-point  arith_type="Signed  (2's comp)"  n_bits=35  bin_pt=31  float_type=Single  exp_bits=8  fraction_bits=24  quantization="Round  (unbiased: +/- Inf)"  overflow=Saturate  en=off  latency=3  dbl_ovrd=off  pipeline=off  block_type=convert
  E[|X-m_x|^2]^2 : Outport
  wires:
  Sub/1 -> square_conv_25bit/1, square_conv_35bit/1
  round_den/1 -> E[|X-m_x|^2]^2/1
  square/1 -> round_den/1
  square_conv_25bit/1 -> square/2
  square_conv_35bit/1 -> square/1
  |m_x|^2/1 -> Sub/2
  E[|X|^2]/1 -> Sub/1

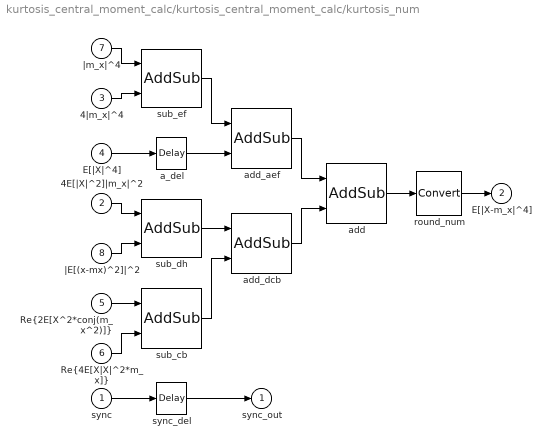
== system kurtosis_central_moment_calc/kurtosis_central_moment_calc/kurtosis_num ==
  sync : Inport
  4E[|X|^2]|m_x|^2 : Inport  Port=2
  4|m_x|^4 : Inport  Port=3
  E[|X|^4] : Inport  Port=4
  "Re{2E[X^2*conj(m_x^2)]}" : Inport  Port=5
  "Re{4E[X|X|^2*m_x]}" : Inport  Port=6
  |m_x|^4 : Inport  Port=7
  |E[(x-mx)^2]|^2 : Inport  Port=8
  a_del : xbsIndex_r4/Delay  rst=off  infoeditControl=Selection of Reset will increase slice count due to use of real FFs and instead of SRLs  en=off  latency=4  dbl_ovrd=off  reg_retiming=off  block_type=delay
  add : xbsIndex_r4/AddSub  mode=Addition  use_carryin=off  use_carryout=off  en=off  latency=4  precision=Full  arith_type="Signed  (2's comp)"  n_bits=36  bin_pt=34  quantization=Truncate  overflow=Wrap  dbl_ovrd=off  use_behavioral_HDL=off  hw_selection=Fabric  pipelined=off  block_type=addsub
  add_aef : xbsIndex_r4/AddSub  mode=Addition  use_carryin=off  use_carryout=off  en=off  latency=4  precision=Full  arith_type="Signed  (2's comp)"  n_bits=36  bin_pt=34  quantization=Truncate  overflow=Wrap  dbl_ovrd=off  use_behavioral_HDL=off  hw_selection=Fabric  pipelined=off  block_type=addsub
  add_dcb : xbsIndex_r4/AddSub  mode=Addition  use_carryin=off  use_carryout=off  en=off  latency=4  precision=Full  arith_type="Signed  (2's comp)"  n_bits=36  bin_pt=34  quantization=Truncate  overflow=Wrap  dbl_ovrd=off  use_behavioral_HDL=off  hw_selection=Fabric  pipelined=off  block_type=addsub
  round_num : xbsIndex_r4/Convert  gui_display_data_type=Fixed-point  arith_type="Signed  (2's comp)"  n_bits=96  bin_pt=84  float_type=Single  exp_bits=8  fraction_bits=24  quantization="Round  (unbiased: +/- Inf)"  overflow=Saturate  en=off  latency=1  dbl_ovrd=off  pipeline=off  block_type=convert
  sub_cb : xbsIndex_r4/AddSub  mode=Subtraction  use_carryin=off  use_carryout=off  en=off  latency=4  precision=Full  arith_type="Signed  (2's comp)"  n_bits=36  bin_pt=34  quantization=Truncate  overflow=Wrap  dbl_ovrd=off  use_behavioral_HDL=off  hw_selection=Fabric  pipelined=off  block_type=addsub
  sub_dh : xbsIndex_r4/AddSub  mode=Subtraction  use_carryin=off  use_carryout=off  en=off  latency=4  precision=Full  arith_type="Signed  (2's comp)"  n_bits=36  bin_pt=34  quantization=Truncate  overflow=Wrap  dbl_ovrd=off  use_behavioral_HDL=off  hw_selection=Fabric  pipelined=off  block_type=addsub
  sub_ef : xbsIndex_r4/AddSub  mode=Subtraction  use_carryin=off  use_carryout=off  en=off  latency=4  precision=Full  arith_type="Signed  (2's comp)"  n_bits=36  bin_pt=34  quantization=Truncate  overflow=Wrap  dbl_ovrd=off  use_behavioral_HDL=off  hw_selection=Fabric  pipelined=off  block_type=addsub
  sync_del : xbsIndex_r4/Delay  rst=off  infoeditControl=Selection of Reset will increase slice count due to use of real FFs and instead of SRLs  en=off  latency=13  dbl_ovrd=off  reg_retiming=off  block_type=delay
  sync_out : Outport
  E[|X-m_x|^4] : Outport  Port=2
  wires:
  sync_del/1 -> sync_out/1
  round_num/1 -> E[|X-m_x|^4]/1
  add/1 -> round_num/1
  add_dcb/1 -> add/2
  add_aef/1 -> add/1
  sub_cb/1 -> add_dcb/2
  sub_dh/1 -> add_dcb/1
  a_del/1 -> add_aef/2
  sub_ef/1 -> add_aef/1
  E[|X|^4]/1 -> a_del/1
  |E[(x-mx)^2]|^2/1 -> sub_dh/2
  4E[|X|^2]|m_x|^2/1 -> sub_dh/1
  "Re{4E[X|X|^2*m_x]}"/1 -> sub_cb/2
  "Re{2E[X^2*conj(m_x^2)]}"/1 -> sub_cb/1
  4|m_x|^4/1 -> sub_ef/2
  |m_x|^4/1 -> sub_ef/1
  sync/1 -> sync_del/1

== system kurtosis_central_moment_calc/kurtosis_central_moment_calc/to_workspace_real ==
  sync_out : Inport
  gateway : xbsIndex_r4/Gateway Out  inherit_from_input=on  hdl_port=off  timing_constraint=None  locs_specified=off  LOCs={}  UseAsDAC=off  DACChannel='1'  block_type=gatewayout
  workspace_input : ToWorkspace  VariableName=sync_out  SampleTime=-1
  _o : Outport
  wires:
  sync_out/1 -> gateway/1, _o/1
  gateway/1 -> workspace_input/1

== system kurtosis_central_moment_calc/kurtosis_central_moment_calc/to_workspace_real1 ==
  d : Inport
  gateway : xbsIndex_r4/Gateway Out  inherit_from_input=on  hdl_port=off  timing_constraint=None  locs_specified=off  LOCs={}  UseAsDAC=off  DACChannel='1'  block_type=gatewayout
  workspace_input : ToWorkspace  VariableName=d  SampleTime=-1
  _o : Outport
  wires:
  d/1 -> gateway/1, _o/1
  gateway/1 -> workspace_input/1

== system kurtosis_central_moment_calc/kurtosis_central_moment_calc/to_workspace_real2 ==
  f : Inport
  gateway : xbsIndex_r4/Gateway Out  inherit_from_input=on  hdl_port=off  timing_constraint=None  locs_specified=off  LOCs={}  UseAsDAC=off  DACChannel='1'  block_type=gatewayout
  workspace_input : ToWorkspace  VariableName=f  SampleTime=-1
  _o : Outport
  wires:
  f/1 -> gateway/1, _o/1
  gateway/1 -> workspace_input/1

== system kurtosis_central_moment_calc/kurtosis_central_moment_calc/to_workspace_real3 ==
  a : Inport
  gateway : xbsIndex_r4/Gateway Out  inherit_from_input=on  hdl_port=off  timing_constraint=None  locs_specified=off  LOCs={}  UseAsDAC=off  DACChannel='1'  block_type=gatewayout
  workspace_input : ToWorkspace  VariableName=a  SampleTime=-1
  _o : Outport
  wires:
  a/1 -> gateway/1, _o/1
  gateway/1 -> workspace_input/1

== system kurtosis_central_moment_calc/kurtosis_central_moment_calc/to_workspace_real4 ==
  c : Inport
  gateway : xbsIndex_r4/Gateway Out  inherit_from_input=on  hdl_port=off  timing_constraint=None  locs_specified=off  LOCs={}  UseAsDAC=off  DACChannel='1'  block_type=gatewayout
  workspace_input : ToWorkspace  VariableName=c  SampleTime=-1
  _o : Outport
  wires:
  c/1 -> gateway/1, _o/1
  gateway/1 -> workspace_input/1

== system kurtosis_central_moment_calc/kurtosis_central_moment_calc/to_workspace_real5 ==
  b : Inport
  gateway : xbsIndex_r4/Gateway Out  inherit_from_input=on  hdl_port=off  timing_constraint=None  locs_specified=off  LOCs={}  UseAsDAC=off  DACChannel='1'  block_type=gatewayout
  workspace_input : ToWorkspace  VariableName=b  SampleTime=-1
  _o : Outport
  wires:
  b/1 -> gateway/1, _o/1
  gateway/1 -> workspace_input/1

== system kurtosis_central_moment_calc/kurtosis_central_moment_calc/to_workspace_real6 ==
  e : Inport
  gateway : xbsIndex_r4/Gateway Out  inherit_from_input=on  hdl_port=off  timing_constraint=None  locs_specified=off  LOCs={}  UseAsDAC=off  DACChannel='1'  block_type=gatewayout
  workspace_input : ToWorkspace  VariableName=e  SampleTime=-1
  _o : Outport
  wires:
  e/1 -> gateway/1, _o/1
  gateway/1 -> workspace_input/1

== system kurtosis_central_moment_calc/kurtosis_central_moment_calc/to_workspace_real7 ==
  third_term : Inport
  gateway : xbsIndex_r4/Gateway Out  inherit_from_input=on  hdl_port=off  timing_constraint=None  locs_specified=off  LOCs={}  UseAsDAC=off  DACChannel='1'  block_type=gatewayout
  workspace_input : ToWorkspace  VariableName=third_term  SampleTime=-1
  _o : Outport
  wires:
  third_term/1 -> gateway/1, _o/1
  gateway/1 -> workspace_input/1
